simulink model "Vending_1"  (R2019a)
settings: Solver=VariableStepAuto  StartTime=0.0  StopTime=60  RelTol=1e-3
settings Model: EnablePacing=on  Creator=kedar  LastModifiedBy=kedar

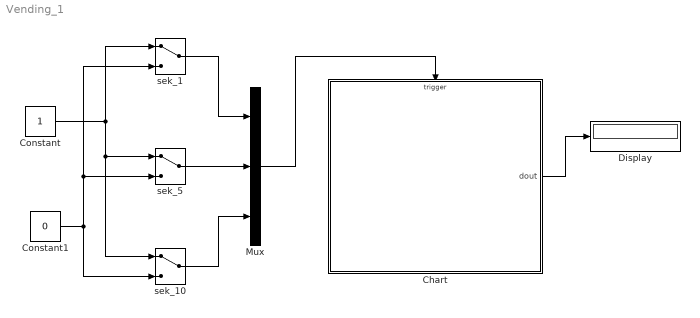
== system Vending_1 ==
  Chart : Stateflow chart  BlockKeywords=__PRM__SERIALIZED__DATA__:Stateflow Chart,Stateflow Diagram  TreatAsAtomicUnit=on
  Constant : Constant
  Constant1 : Constant  Value=0
  Display : Display
  Mux : Mux  Inputs=3
  sek_1 : ManualSwitch
  sek_10 : ManualSwitch
  sek_5 : ManualSwitch
  wires:
  Constant/1 -> sek_10/1, sek_5/1, sek_1/1
  Constant1/1 -> sek_10/2, sek_5/2, sek_1/2
  Mux/1 -> Chart/Trigger
  sek_1/1 -> Mux/1
  sek_5/1 -> Mux/2
  sek_10/1 -> Mux/3
  Chart/1(dout) -> Display/1

== stateflow chart Vending_1/Chart ==
  settings: executeAtInitialization=1
  state VendingMachine
    en: money = 0;
    state MoneyCollector
      on sek_1: money = money + 1;
      dout = money
      on sek_5: money = money + 5;
      dout = money
      on sek_10: money = money + 10;
      dout = money
    state SnackVendor
      if(money<6){
      printf["Put more money!!!"]
      )
      elseif (money>=6){
      snack1
      }
    (default) -> MoneyCollector
    MoneyCollector -> SnackVendor : [money>=6]
  (default) -> VendingMachine
  data: money local; dout output
  events: sek_1 input RISING_EDGE_EVENT; sek_5 input RISING_EDGE_EVENT; sek_10 input RISING_EDGE_EVENT
